simulink model "Model_vertical_lqi_fuzzy"  (R2015a)
settings: Solver=ode4  StartTime=0.0  StopTime=50  FixedStep=1e-3  RelTol=1e-3
undefined symbols (not defined in the file or in its folder): a, alpha_0, f_v, I_v, J_v, K_lqi, L, lin_A, lin_alpha_v, lin_B, lin_C, lin_u_v, lin_velocity_v, lin_w_v, sigbuilder_block, wsp_M_V, wsp_U_V
libraries: fuzblock x1
settings Model: Creator=Student  LastModifiedBy=Student

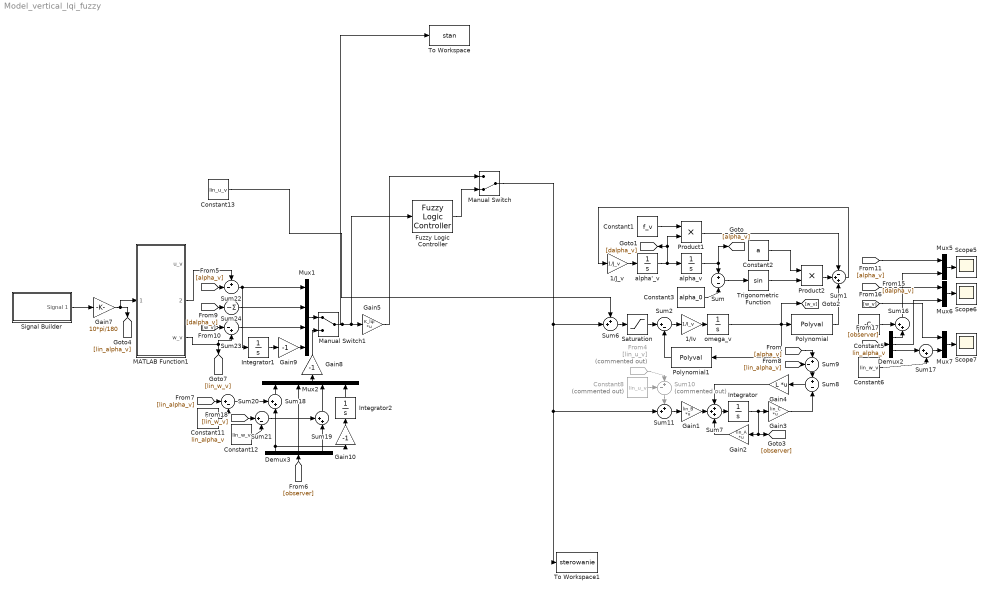
== system Model_vertical_lqi_fuzzy ==
  1/Iv : Gain  Gain=1/I_v
  1/J_v : Gain  Gain=1/J_v
  Constant1 : Constant  Value=f_v
  Constant11 : Constant  Value=lin_alpha_v
  Constant12 : Constant  Value=lin_w_v
  Constant13 : Constant  Value=lin_u_v
  Constant2 : Constant  Value=a
  Constant3 : Constant  Value=alpha_0
  Constant5 : Constant  Value=lin_alpha_v
  Constant6 : Constant  Value=lin_w_v
  Constant8 : Constant  Commented=on  Value=lin_u_v
  Demux2 : Demux  Outputs=3
  Demux3 : Demux  Outputs=3
  From4 : From  Commented=on  GotoTag=lin_u_v
  Fuzzy Logic Controller : fuzblock/Fuzzy Logic  Controller  fis=fis
  Gain1 : Gain  Gain=lin_B  Multiplication=Matrix(K*u)
  Gain10 : Gain  Gain=-1
  Gain2 : Gain  Gain=lin_A  Multiplication=Matrix(K*u)
  Gain3 : Gain  Gain=lin_C  Multiplication=Matrix(K*u)
  Gain4 : Gain  Gain=L  Multiplication=Matrix(K*u)
  Gain5 : Gain  Gain=K_lqi  Multiplication=Matrix(K*u)
  Gain7 : Gain  Gain=10*pi/180
  Gain8 : Gain  Gain=-1
  Gain9 : Gain  Gain=-1
  Integrator : Integrator  InitialCondition=[0;0;0]
  Integrator1 : Integrator
  Integrator2 : Integrator
  MATLAB Function1 : MATLAB Function  TreatAsAtomicUnit=on
  Manual Switch : ManualSwitch  CurrentSetting=0
  Manual Switch1 : ManualSwitch
  Mux1 : Mux
  Mux2 : Mux
  Mux5 : Mux  Inputs=2
  Mux6 : Mux  Inputs=2
  Mux7 : Mux  Inputs=2
  Polynomial : Polyval  Coefs=wsp_M_V
  Polynomial1 : Polyval  Coefs=wsp_U_V
  Product1 : Product
  Product2 : Product
  Saturation : Saturate  UpperLimit=1  LowerLimit=-1
  Scope5 : Scope
      settings: YMin=-0.4  YMax=0.3
  Scope6 : Scope
      settings: YMin=-0.06773  YMax=0.05947  SaveName=ScopeData2
  Scope7 : Scope
      settings: YMin=171.46242  YMax=188.98603  SaveName=ScopeData3
  Signal Builder : Subsystem  Tag=STV Subsys  LoadFcn=sigbuilder_block('load');  StartFcn=sigbuilder_block('start');  StopFcn=sigbuilder_block('stop');  ClipboardFcn=sigbuilder_block('clipboard');  mask(Sigbuilder block){}
      mask help: Simulink:masks:SigbuilderBlock_MD
      mask init:
      | if ~strcmp(get_param(bdroot(gcbh),'SimulationStatus'),'stopped') tuvar = sigbuilder_block('maskInit'); end
      settings: CopyFcn=sigbuilder_block('copy');  DeleteFcn=sigbuilder_block('delete');  ModelCloseFcn=sigbuilder_block('modelClose');  PreSaveFcn=sigbuilder_block('preSave');  PauseFcn=sigbuilder_block('pause');  ContinueFcn=sigbuilder_block('continue');  NameChangeFcn=sigbuilder_block('namechange');  OpenFcn=sigbuilder_block('open',[437.6 199.2 550.4 400 ]);  CloseFcn=sigbuilder_block('close');
      mask Display: plot(0, 0, 100, 100,[2, 2, 32, 32, 2], [68, 8, 8, 68, 68],[32, 2], [38, 38], [32, 19, 2],[53, 60, 44], [32, 17, 17, 2],[16, 16, 31, 31]);txt = getActiveGroup(gcbh);text(2, 100, txt,'verticalAlignment', 'top');
  Sum : Sum  Inputs=+|-
  Sum1 : Sum  Inputs=-++
  Sum10 : Sum  Commented=on  Inputs=-+|
  Sum{6,11,16,18..19} (5 alike) : Sum  Inputs=++|
  Sum17 : Sum  Inputs=|++
  Sum2 : Sum  Inputs=|+-
  Sum20 : Sum  Inputs=|+-
  Sum21 : Sum  Inputs=|+-
  Sum22 : Sum  Inputs=+-|
  Sum23 : Sum  Inputs=|-+
  Sum24 : Sum  Inputs=|-|
  Sum7 : Sum  Inputs=+++
  Sum8 : Sum  Inputs=+|-
  Sum9 : Sum  Inputs=-+|
  To Workspace : ToWorkspace  VariableName=stan  SaveFormat=Timeseries  SampleTime=-1
  To Workspace1 : ToWorkspace  VariableName=sterowanie  SaveFormat=Timeseries  SampleTime=-1
  Trigonometric Function : Trigonometry
  alpha'_v : Integrator  InitialCondition=lin_velocity_v
  alpha_v : Integrator  InitialCondition=lin_alpha_v+0.1
  omega_v : Integrator  InitialCondition=lin_w_v
  wires:
  omega_v/1 -> [w_v], Polynomial1/1, Polynomial/1
  Product2/1 -> Sum1/2
  Sum2/1 -> 1/Iv/1
  Sum/1 -> Trigonometric Function/1
  Constant3/1 -> Sum/2
  Constant1/1 -> Product1/1
  alpha_v/1 -> [alpha_v], Sum/1
  Constant2/1 -> Product2/1
  Polynomial/1 -> Sum1/3
  Sum1/1 -> 1/J_v/1
  Product1/1 -> Sum1/1
  1/J_v/1 -> alpha'_v/1
  alpha'_v/1 -> [dalpha_v], Product1/2, alpha_v/1
  Trigonometric Function/1 -> Product2/2
  Polynomial1/1 -> Sum2/2
  1/Iv/1 -> omega_v/1
  [alpha_v] -> Sum9/2
  Sum6/1 -> Saturation/1
  Saturation/1 -> Sum2/1
  Gain1/1 -> Sum7/2
  Sum7/1 -> Integrator/1
  Gain2/1 -> Sum7/3
  Integrator/1 -> Gain3/1, [observer], Gain2/1
  Gain3/1 -> Sum8/2
  Sum8/1 -> Gain4/1
  Gain4/1 -> Sum7/1
  Gain7/1 -> [lin_alpha_v], MATLAB Function1/1(alpha_vin)
  Sum9/1 -> Sum8/1
  [lin_alpha_v] -> Sum9/1
  [dalpha_v] -> Mux6/1
  Sum16/1 -> Mux5/2
  Mux7/1 -> Scope7/1
  Demux2/3 -> Sum17/1
  Mux5/1 -> Scope5/1
  Demux2/1 -> Sum16/2
  Sum17/1 -> Mux7/2
  Mux6/1 -> Scope6/1
  [observer] -> Demux2/1
  Constant6/1 -> Sum17/2
  [w_v] -> Mux7/1
  Demux2/2 -> Mux6/2
  Constant5/1 -> Sum16/1
  [alpha_v] -> Mux5/1
  Sum11/1 -> Gain1/1
  Sum10/1 -> Sum11/1
  From4/1 -> Sum10/2
  Constant8/1 -> Sum10/1
  Signal Builder/1(Signal 1) -> Gain7/1
  [alpha_v] -> Sum22/2
  Sum22/1 -> Mux1/1, Integrator1/1
  MATLAB Function1/2(alpha_v) -> Sum22/1
  Sum23/1 -> Mux1/3
  [w_v] -> Sum23/1
  MATLAB Function1/3(w_v) -> Sum23/2, [lin_w_v]
  [dalpha_v] -> Sum24/1
  Sum24/1 -> Mux1/2
  Manual Switch1/1 -> To Workspace/1, Fuzzy Logic Controller/1, Gain5/1
  Mux1/1 -> Manual Switch1/1
  Demux3/3 -> Sum19/2
  Gain8/1 -> Manual Switch1/2
  Integrator1/1 -> Gain9/1
  Gain9/1 -> Mux1/4
  Demux3/2 -> Mux2/2
  Demux3/1 -> Gain10/1, Sum18/2
  Integrator2/1 -> Mux2/4
  Gain10/1 -> Integrator2/1
  [observer] -> Demux3/1
  Mux2/1 -> Gain8/1
  Sum18/1 -> Mux2/1
  Sum19/1 -> Mux2/3
  [lin_alpha_v] -> Sum20/1
  Sum20/1 -> Sum18/1
  Constant11/1 -> Sum20/2
  Sum21/1 -> Sum19/1
  [lin_w_v] -> Sum21/1
  Constant12/1 -> Sum21/2
  Constant13/1 -> Sum6/1
  Fuzzy Logic Controller/1 -> Manual Switch/2
  Gain5/1 -> Manual Switch/1
  Manual Switch/1 -> To Workspace1/1, Sum11/2, Sum6/2

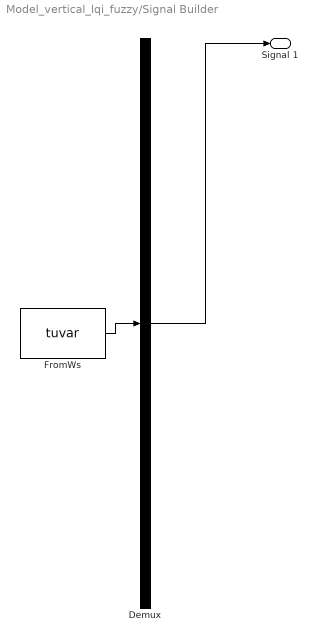
== system Model_vertical_lqi_fuzzy/Signal Builder ==
  Demux : Demux  Tag=STV Demux  Outputs=1
  FromWs : FromWorkspace  Tag=STV FromWs  VariableName=tuvar  SampleTime=0
      SigBuilderData=|
      | common.afterFinalStr = 'Extrapolate'
      | common.sampleTime = 0
      | dataSet.timeRange = [0 50]
      | dataSet.name = 'Group 1'
      | sbobj.Groups.Name = 'Group 1'
      | sbobj.Groups.Signals.Name = 'Signal 1'
      | sbobj.Groups.Signals.XData = [0 2 4 5 5 10 10 20 20 30.1 30.1 40 40 50]
      | sbobj.Groups.Signals.YData = [-0.01 -0.01 -0.01 -0.01 -1 -1 1 1 0 0 -1 -1 0 0]
      | sbobj.Groups.TimeRange = [0 50]
  Signal 1 : Outport  Tag=STV Outport
  wires:
  Demux/1 -> Signal 1/1
  FromWs/1 -> Demux/1

== matlab function Model_vertical_lqi_fuzzy/MATLAB Function1 ==
  data: u_v output double size=1 [0..1]; alpha_vin input; alpha_v output; w_v output double size=1
function [u_v, alpha_v, w_v] = Lin(alpha_vin)

const = load('Lin_simulink_test.mat');

w_v = roots(const.wsp_M_V+[zeros(1,length(const.wsp_M_V)-1) const.a*sin(alpha_vin-const.alpha_0)]);
w_v = real(w_v(w_v>-350 & w_v<350 & imag(w_v)==0));
w_v = w_v(1);
u_v = polyval(const.wsp_U_V, w_v);
u_v = u_v(1);
alpha_v = alpha_vin;
